simulink model "sundaresan_krishnaswami"  (R2018a)
settings: Solver=VariableStepAuto  StartTime=0.0  StopTime=30  RelTol=1e-3
libraries: simulink x1
settings Model: Creator=Diego  LastModifiedBy=Diego

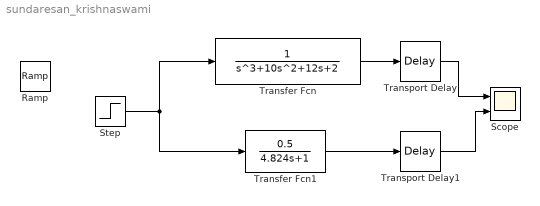
== system sundaresan_krishnaswami ==
  Scope : Scope  NumInputPorts=2
  Step : Step  Time=0  SampleTime=0
  Transfer Fcn : TransferFcn  Denominator=[1 10 12 2]
  Transfer Fcn1 : TransferFcn  Numerator=[0.5]  Denominator=[4.824 1]
  Transport Delay : TransportDelay  DelayTime=3
  Transport Delay1 : TransportDelay  DelayTime=4.27
  Ramp : simulink/Sources/Ramp  IOType=siggen  slope=1  start=0  InitialOutput=0
  wires:
  Transfer Fcn1/1 -> Transport Delay1/1
  Transfer Fcn/1 -> Transport Delay/1
  Transport Delay/1 -> Scope/1
  Transport Delay1/1 -> Scope/2
  Step/1 -> Transfer Fcn1/1, Transfer Fcn/1
